simulink model "comparacion_fuzzy_pid"  (R2020b)
settings: Solver=FixedStepAuto  StartTime=0.0  StopTime=10  FixedStep=0.01  RelTol=1e-3
values from neighbouring files (symbols this model uses):
  C0 = 1/(C*Ce*(tauC+L/2))    (= 4.44444444444)    [comparacion_controladores.m]
  C1 = max(T,L/2)*C0    [comparacion_controladores.m]
  Cd = min(T,L/2)*Ce    [comparacion_controladores.m]
  Ce = 1    [comparacion_controladores.m]
  pidController = pidtune(G,'pidf')    [comparacion_controladores.m]
libraries: cstblocks x3, fuzblock x2
settings Model: Creator=The MathWorks, Inc.  LastModifiedBy=snopv
settings DebuggingCC: SymbolicDimsDataTypeCodeGenerationDiagnostic=none

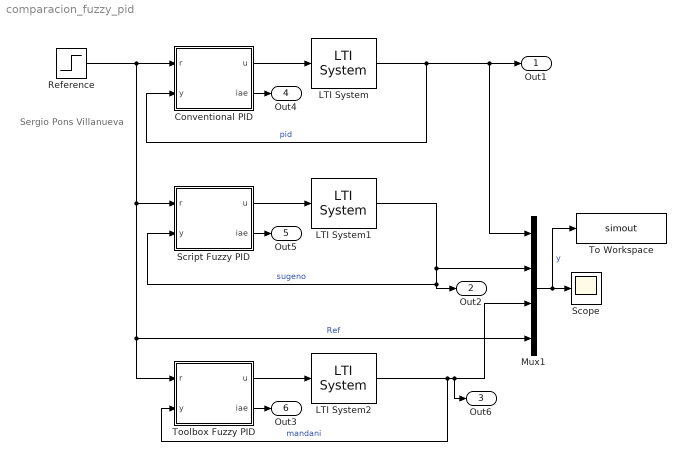
== system comparacion_fuzzy_pid ==
  note: Sergio Pons Villanueva
  Conventional PID : Subsystem
  LTI System : cstblocks/LTI System  sys=G  IC=[]
  LTI System1 : cstblocks/LTI System  sys=G  IC=[]
  LTI System2 : cstblocks/LTI System  sys=G  IC=[]
  Mux1 : Mux
  Reference : Step  SampleTime=0
  Scope : Scope
  Script Fuzzy PID : Subsystem
  To Workspace : ToWorkspace  VariableName=simout  SaveFormat=Timeseries  SampleTime=-1
  Toolbox Fuzzy PID : Subsystem
  Out1 : Outport  VectorParamsAs1DForOutWhenUnconnected=off
  Out2 : Outport  Port=2  VectorParamsAs1DForOutWhenUnconnected=off
  Out6 : Outport  Port=3  VectorParamsAs1DForOutWhenUnconnected=off
  Out4 : Outport  Port=4  VectorParamsAs1DForOutWhenUnconnected=off
  Out5 : Outport  Port=5  VectorParamsAs1DForOutWhenUnconnected=off
  Out3 : Outport  Port=6  VectorParamsAs1DForOutWhenUnconnected=off
  wires:
  Mux1/1 -> To Workspace/1, Scope/1  "y"
  LTI System/1 -> Mux1/1, Out1/1, Conventional PID/2(y)  "pid"
  Conventional PID/1(u) -> LTI System/1
  Script Fuzzy PID/1(u) -> LTI System1/1
  LTI System1/1 -> Out2/1, Script Fuzzy PID/2(y), Mux1/2  "sugeno"
  Conventional PID/2(iae) -> Out4/1
  Script Fuzzy PID/2(iae) -> Out5/1
  Reference/1 -> Mux1/4, Toolbox Fuzzy PID/1(r), Script Fuzzy PID/1(r), Conventional PID/1(r)  "Ref"
  Toolbox Fuzzy PID/2(iae) -> Out3/1
  LTI System2/1 -> Toolbox Fuzzy PID/2(y), Out6/1, Mux1/3  "mandani"
  Toolbox Fuzzy PID/1(u) -> LTI System2/1

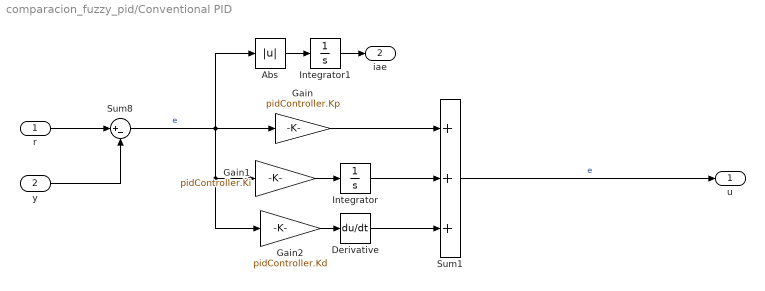
== system comparacion_fuzzy_pid/Conventional PID ==
  r : Inport
  y : Inport  Port=2
  Abs : Abs
  Derivative : Derivative  CoefficientInTFapproximation=pidController.Tf
  Gain : Gain  Gain=pidController.Kp
  Gain1 : Gain  Gain=pidController.Ki
  Gain2 : Gain  Gain=pidController.Kd
  Integrator : Integrator
  Integrator1 : Integrator
  Sum1 : Sum  Inputs=+++
  Sum8 : Sum  Inputs=|+-
  u : Outport  VectorParamsAs1DForOutWhenUnconnected=off
  iae : Outport  Port=2  VectorParamsAs1DForOutWhenUnconnected=off
  wires:
  r/1 -> Sum8/1
  y/1 -> Sum8/2
  Sum1/1 -> u/1  "e"
  Sum8/1 -> Abs/1, Gain2/1, Gain1/1, Gain/1  "e"
  Gain/1 -> Sum1/1
  Gain1/1 -> Integrator/1
  Integrator/1 -> Sum1/2
  Gain2/1 -> Derivative/1
  Derivative/1 -> Sum1/3
  Abs/1 -> Integrator1/1
  Integrator1/1 -> iae/1

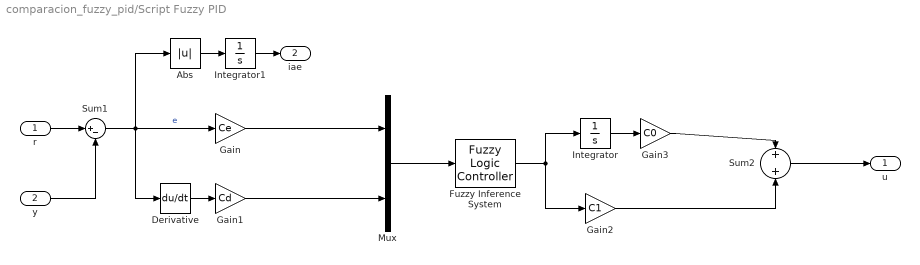
== system comparacion_fuzzy_pid/Script Fuzzy PID ==
  r : Inport
  y : Inport  Port=2
  Abs : Abs
  Derivative : Derivative  CoefficientInTFapproximation=1
  Fuzzy Inference System : fuzblock/Fuzzy Logic  Controller  FIS=fis1  OutputSampleNumber=101  DataType=double  FuzzifiedInputs=off  RuleFiringStrengths=off  RuleOutputs=off  AggregatedOutputs=off  SimulateUsing=Code generation  OutOfRangeInputValueMessage=none  NoRuleFiredMessage=none  EmptyOutputFuzzySetMessage=none
  Gain : Gain  Gain=Ce
  Gain1 : Gain  Gain=Cd
  Gain2 : Gain  Gain=C1
  Gain3 : Gain  Gain=C0
  Integrator : Integrator
  Integrator1 : Integrator
  Mux : Mux  Inputs=2
  Sum1 : Sum  Inputs=|+-
  Sum2 : Sum  Inputs=+|+
  u : Outport  VectorParamsAs1DForOutWhenUnconnected=off
  iae : Outport  Port=2  VectorParamsAs1DForOutWhenUnconnected=off
  wires:
  Sum1/1 -> Abs/1, Derivative/1, Gain/1  "e"
  Mux/1 -> Fuzzy Inference System/1
  Fuzzy Inference System/1 -> Gain2/1, Integrator/1
  r/1 -> Sum1/1
  y/1 -> Sum1/2
  Sum2/1 -> u/1
  Derivative/1 -> Gain1/1
  Integrator/1 -> Gain3/1
  Gain/1 -> Mux/1
  Gain1/1 -> Mux/2
  Gain2/1 -> Sum2/2
  Gain3/1 -> Sum2/1
  Abs/1 -> Integrator1/1
  Integrator1/1 -> iae/1

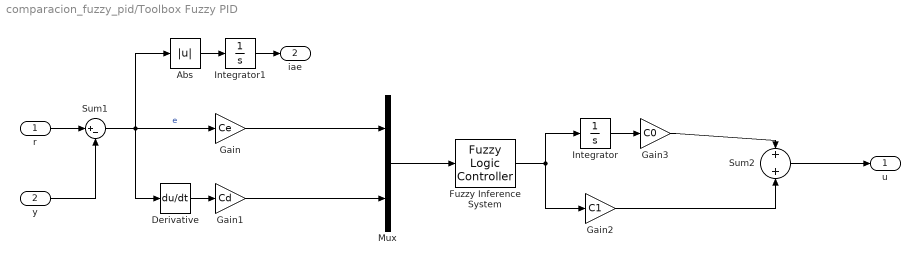
== system comparacion_fuzzy_pid/Toolbox Fuzzy PID ==
  r : Inport
  y : Inport  Port=2
  Abs : Abs
  Derivative : Derivative  CoefficientInTFapproximation=1
  Fuzzy Inference System : fuzblock/Fuzzy Logic  Controller  FIS=fismandani  OutputSampleNumber=101  DataType=double  FuzzifiedInputs=off  RuleFiringStrengths=off  RuleOutputs=off  AggregatedOutputs=off  SimulateUsing=Code generation  OutOfRangeInputValueMessage=none  NoRuleFiredMessage=none  EmptyOutputFuzzySetMessage=none
  Gain : Gain  Gain=Ce
  Gain1 : Gain  Gain=Cd
  Gain2 : Gain  Gain=C1
  Gain3 : Gain  Gain=C0
  Integrator : Integrator
  Integrator1 : Integrator
  Mux : Mux  Inputs=2
  Sum1 : Sum  Inputs=|+-
  Sum2 : Sum  Inputs=+|+
  u : Outport  VectorParamsAs1DForOutWhenUnconnected=off
  iae : Outport  Port=2  VectorParamsAs1DForOutWhenUnconnected=off
  wires:
  Sum1/1 -> Abs/1, Derivative/1, Gain/1  "e"
  Mux/1 -> Fuzzy Inference System/1
  Fuzzy Inference System/1 -> Gain2/1, Integrator/1
  r/1 -> Sum1/1
  y/1 -> Sum1/2
  Sum2/1 -> u/1
  Derivative/1 -> Gain1/1
  Integrator/1 -> Gain3/1
  Gain/1 -> Mux/1
  Gain1/1 -> Mux/2
  Gain2/1 -> Sum2/2
  Gain3/1 -> Sum2/1
  Abs/1 -> Integrator1/1
  Integrator1/1 -> iae/1
